simulink model "prob2"  (R2020a)
settings: Solver=VariableStepAuto  StartTime=0.0  StopTime=120  RelTol=1e-3
values from neighbouring files (symbols this model uses):
  b = 50.0    [dict.sldd]
  m = 1000.0    [dict.sldd]
undefined symbols (not defined in the file or in its folder): ki, kp
settings Model: DataDictionary=dict.sldd  Creator=I3  LastModifiedBy=I3

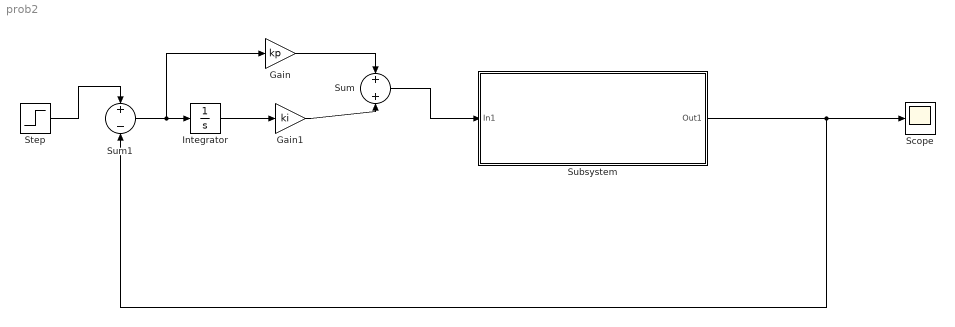
== system prob2 ==
  Gain : Gain  Gain=kp
  Gain1 : Gain  Gain=ki
  Integrator : Integrator
  Scope : Scope
  Step : Step  After=u  SampleTime=0
  Subsystem : Subsystem
  Sum : Sum
  Sum1 : Sum  Inputs=+-
  wires:
  Sum/1 -> Subsystem/1(In1)
  Subsystem/1(Out1) -> Sum1/2, Scope/1
  Integrator/1 -> Gain1/1
  Sum1/1 -> Gain/1, Integrator/1
  Gain/1 -> Sum/1
  Gain1/1 -> Sum/2
  Step/1 -> Sum1/1

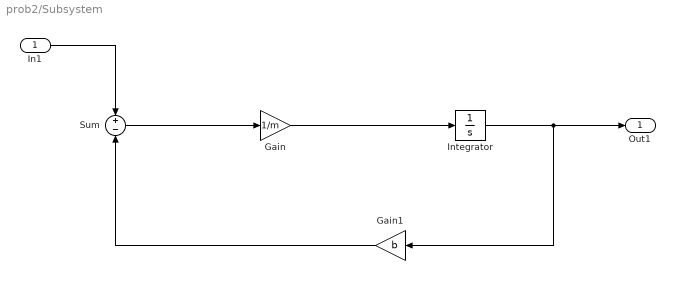
== system prob2/Subsystem ==
  In1 : Inport
  Gain : Gain  Gain=1/m
  Gain1 : Gain  Gain=b
  Integrator : Integrator
  Sum : Sum  Inputs=+-
  Out1 : Outport
  wires:
  Gain1/1 -> Sum/2
  Integrator/1 -> Out1/1, Gain1/1
  Sum/1 -> Gain/1
  Gain/1 -> Integrator/1
  In1/1 -> Sum/1
